simulink model "Testing"  (R2025b)
settings: Solver=VariableStepAuto  StartTime=0.0  StopTime=10.0  RelTol=1e-3
settings Model: Creator=jwjar  LastModifiedBy=jwjar

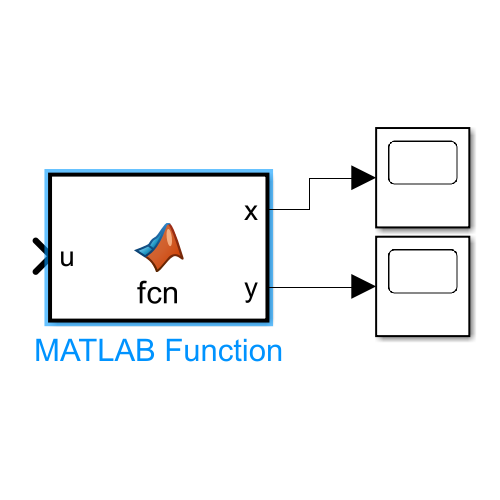
[thumbnail: Simulink's stored preview of the top-level diagram]
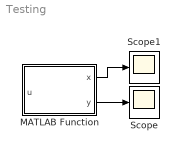
== system Testing ==
  MATLAB Function : MATLAB Function  TreatAsAtomicUnit=on
  Scope : Scope
      settings: ActiveDisplayYMinimum=1  ActiveDisplayYMaximum=3
  Scope1 : Scope
      settings: ActiveDisplayYMinimum=0.9  ActiveDisplayYMaximum=1.1
  wires:
  MATLAB Function/2(y) -> Scope/1
  MATLAB Function/1(x) -> Scope1/1

== matlab function Testing/MATLAB Function ==
  data: x output; u input; y output
function [x, y]= fcn(u)
x = 0.0;
y = 0.0;
coder.extrinsic("py.compare_agents.testing")
position = double(py.compare_agents.testing());
x = position(1);
y = position(2);
fprintf("x: %f, y: %f\n", x, y)
end
